simulink model "BatterySOCEstimationDeepLearning"  (R2024b)
settings: Solver=FixedStepDiscrete  StartTime=0.0  StopTime=steps  FixedStep=Ts  RelTol=1e-3
undefined symbols (not defined in the file or in its folder): recurrentNet
libraries: dlutilitylib x2, dlconvfclib x2, dlsequencelib x2, dlactivationlib x1
settings Model: ModifiedByFormat=The MathWorks, Inc.  Creator=The MathWorks, Inc.  LastModifiedBy=The MathWorks, Inc.
settings DataIOCC: ExternalInput=ds  LoadExternalInput=on
settings OptimizationCC: DefaultParameterBehavior=Inlined  EnhancedBackFolding=on  PassReuseOutputArgsAs=Individual arguments  ZeroExternalMemoryAtStartup=off  ZeroInternalMemoryAtStartup=off  OptimizeBlockOrder=speed  DifferentSizesBufferReuse=on  OptimizationCustomize=off  EfficientTunableParamExpr=on
settings DebuggingCC: ParameterTunabilityLossMsg=error
settings SFSimCC: MATLABDynamicMemAlloc=off
settings RTWCC: Description=Embedded Coder  SystemTargetFile=ert.tlc  TemplateMakefile=ert_default_tmf
settings CodeAppCC: ForceParamTrailComments=on  IgnoreCustomStorageClasses=off  OperatorAnnotations=on  SimulinkDataObjDesc=on  SFDataObjDesc=on  InsertBlockDesc=on
settings ERTTargetCC: TargetLangStandard=C99 (ISO)  GenerateSampleERTMain=on  SupportVariableSizeSignals=on  ERTCustomFileTemplate=example_file_process.tlc

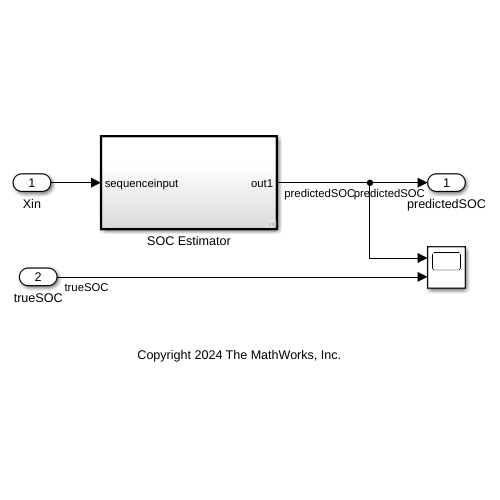
[thumbnail: Simulink's stored preview of the top-level diagram]
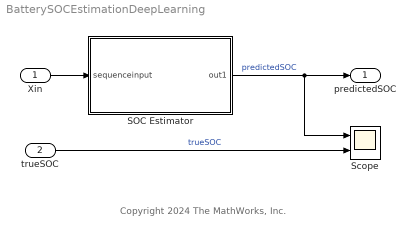
== system BatterySOCEstimationDeepLearning ==
  note: Copyright 2024 The MathWorks, Inc.
  Xin : Inport
  trueSOC : Inport  Port=2
  SOC Estimator : Subsystem  TreatAsAtomicUnit=on
  Scope : Scope  NumInputPorts=2
  predictedSOC : Outport
  wires:
  Xin/1 -> SOC Estimator/1(sequenceinput)
  trueSOC/1 -> Scope/2  "trueSOC"
  SOC Estimator/1(out1) -> predictedSOC/1, Scope/1  "predictedSOC"

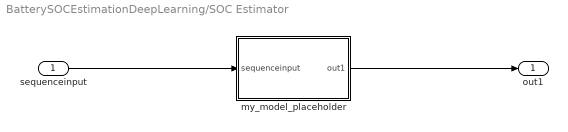
== system BatterySOCEstimationDeepLearning/SOC Estimator ==
  sequenceinput : Inport  PortDimensions="[3  1]"
  my_model_placeholder : Subsystem
  out1 : Outport
  wires:
  my_model_placeholder/1(out1) -> out1/1
  sequenceinput/1 -> my_model_placeholder/1(sequenceinput)

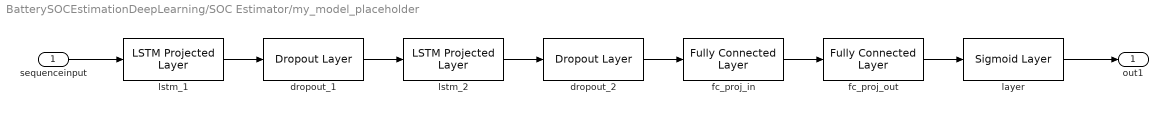
== system BatterySOCEstimationDeepLearning/SOC Estimator/my_model_placeholder ==
  sequenceinput : Inport  PortDimensions="[3  1]"
  dropout_1 : dlutilitylib/Dropout Layer  SampleTime=-1
      settings: LibrarySourceBlock=|
      | hdlsllib/Ports &
      | Subsystems/Subsystem
  dropout_2 : dlutilitylib/Dropout Layer  SampleTime=-1
      settings: LibrarySourceBlock=|
      | hdlsllib/Ports &
      | Subsystems/Subsystem
  fc_proj_in : dlconvfclib/Fully Connected Layer  Layer=recurrentNet.Layers(6)  OutMin=[]  OutMax=[]  WeightsDataTypeStr=Inherit: Inherit via back propagation  WeightsMin=[]  WeightsMax=[]  BiasDataTypeStr=Inherit: Inherit via back propagation  BiasMin=[]  BiasMax=[]  MatrixMultiplyMin=[]  MatrixMultiplyMax=[]  SampleTime=-1
      settings: DataFormat=CT
  fc_proj_out : dlconvfclib/Fully Connected Layer  Layer=recurrentNet.Layers(7)  OutMin=[]  OutMax=[]  WeightsDataTypeStr=Inherit: Inherit via back propagation  WeightsMin=[]  WeightsMax=[]  BiasDataTypeStr=Inherit: Inherit via back propagation  BiasMin=[]  BiasMax=[]  MatrixMultiplyMin=[]  MatrixMultiplyMax=[]  SampleTime=-1
      settings: DataFormat=CT
  layer : dlactivationlib/Sigmoid Layer  ApproximationMethod=None  OutMin=[]  OutMax=[]  OutDataTypeStr=Inherit: Inherit via back propagation  SampleTime=-1
  lstm_1 : dlsequencelib/LSTM Projected Layer  Layer=recurrentNet.Layers(2)  Stateful=on  ApproximationMethod=None  InputWeightsDataTypeStr=Inherit: Inherit via back propagation  InputWeightsMin=[]  InputWeightsMax=[]  RecurrentWeightsDataTypeStr=Inherit: Inherit via back propagation  RecurrentWeightsMin=[]  RecurrentWeightsMax=[]  BiasDataTypeStr=Inherit: Inherit via back propagation  BiasMin=[]  BiasMax=[]  InputProjectorWeightsDataTypeStr=Inherit: Inherit via back propagation  InputProjectorWeightsMin=[]  InputProjectorWeightsMax=[]  OutputProjectorWeightsDataTypeStr=Inherit: Inherit via back propagation  OutputProjectorWeightsMin=[]  OutputProjectorWeightsMax=[]  InitialCellStateDataTypeStr=Inherit: Inherit via back propagation  InitialCellStateMin=[]  InitialCellStateMax=[]  CellStateMin=[]  CellStateMax=[]  InitialHiddenStateDataTypeStr=Inherit: Inherit via back propagation  InitialHiddenStateMin=[]  InitialHiddenStateMax=[]  HiddenStateMin=[]  HiddenStateMax=[]  InputWeightsMatrixMultiplyOutMin=[]  InputWeightsMatrixMultiplyOutMax=[]  RecurrentWeightsMatrixMultiplyOutMin=[]  RecurrentWeightsMatrixMultiplyOutMax=[]  InputProjectorWeightsMatrixMultiplyOutMin=[]  InputProjectorWeightsMatrixMultiplyOutMax=[]  OutputProjectorWeightsMatrixMultiplyOutMin=[]  OutputProjectorWeightsMatrixMultiplyOutMax=[]  LinearGateAddOutMin=[]  LinearGateAddOutMax=[]  CellStateProductOutMin=[]  CellStateProductOutMax=[]  SampleTime=-1
      settings: DataFormat=CT
  lstm_2 : dlsequencelib/LSTM Projected Layer  Layer=recurrentNet.Layers(4)  Stateful=on  ApproximationMethod=None  InputWeightsDataTypeStr=Inherit: Inherit via back propagation  InputWeightsMin=[]  InputWeightsMax=[]  RecurrentWeightsDataTypeStr=Inherit: Inherit via back propagation  RecurrentWeightsMin=[]  RecurrentWeightsMax=[]  BiasDataTypeStr=Inherit: Inherit via back propagation  BiasMin=[]  BiasMax=[]  InputProjectorWeightsDataTypeStr=Inherit: Inherit via back propagation  InputProjectorWeightsMin=[]  InputProjectorWeightsMax=[]  OutputProjectorWeightsDataTypeStr=Inherit: Inherit via back propagation  OutputProjectorWeightsMin=[]  OutputProjectorWeightsMax=[]  InitialCellStateDataTypeStr=Inherit: Inherit via back propagation  InitialCellStateMin=[]  InitialCellStateMax=[]  CellStateMin=[]  CellStateMax=[]  InitialHiddenStateDataTypeStr=Inherit: Inherit via back propagation  InitialHiddenStateMin=[]  InitialHiddenStateMax=[]  HiddenStateMin=[]  HiddenStateMax=[]  InputWeightsMatrixMultiplyOutMin=[]  InputWeightsMatrixMultiplyOutMax=[]  RecurrentWeightsMatrixMultiplyOutMin=[]  RecurrentWeightsMatrixMultiplyOutMax=[]  InputProjectorWeightsMatrixMultiplyOutMin=[]  InputProjectorWeightsMatrixMultiplyOutMax=[]  OutputProjectorWeightsMatrixMultiplyOutMin=[]  OutputProjectorWeightsMatrixMultiplyOutMax=[]  LinearGateAddOutMin=[]  LinearGateAddOutMax=[]  CellStateProductOutMin=[]  CellStateProductOutMax=[]  SampleTime=-1
      settings: DataFormat=CT
  out1 : Outport
  wires:
  fc_proj_in/1 -> fc_proj_out/1
  lstm_2/1 -> dropout_2/1
  dropout_2/1 -> fc_proj_in/1
  fc_proj_out/1 -> layer/1
  sequenceinput/1 -> lstm_1/1
  layer/1 -> out1/1
  lstm_1/1 -> dropout_1/1
  dropout_1/1 -> lstm_2/1
